simulink model "rf"  (R2016a)
settings: Solver=VariableStepAuto  StartTime=0.0  StopTime=10  RelTol=1e-3
values from neighbouring files (symbols this model uses):
  b_low_pass = fir1(low_pass_order, freq2rad(max_stop_freq_fir, fs), 'low', kaiser(low_pass_order+1, 0.5))    [graphs.m]    (also in rf_controller.m)
  band_pass_grpdelay = 10    [rf_controller.m]
  bandpass_a_H = bandpass_a_vec{i+M}    [rf_controller.m]
  bandpass_a_L = bandpass_a_vec{i}    [rf_controller.m]
  bandpass_b_H = bandpass_b_vec{i+M}    [rf_controller.m]
  bandpass_b_L = bandpass_b_vec{i}    [rf_controller.m]
  fs = 4224000    [bandpass_test.m]    (also in graphs.m = 50688000; main.m = 2*max_stop_freq_fir; rf_controller.m = 1/(time(2)-time(1)))
  LO2_sig = cos(2*pi*LO2 * time)    [rf_controller.m]
  low_pass_grpdelay = low_pass_order/2    (= 10)    [graphs.m]    (also in rf_controller.m)
  sig_len_band_pass = length(signal)/64    [rf_controller.m]
  sig_len_low_pass = length(signal)    [rf_controller.m]
undefined symbols (not defined in the file or in its folder): signal
libraries: dspsigops x5, lib1 x2
settings Model: Creator=jbeau  LastModifiedBy=jbeau
settings GRTTargetCC: GeneratePreprocessorConditionals=Use local settings

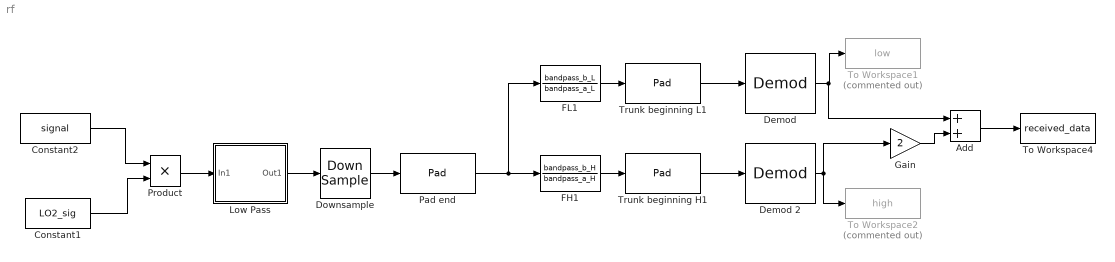
== system rf ==
  Add : Sum  OutDataTypeStr=double
  Constant1 : Constant  Value=LO2_sig  SampleTime=fs
  Constant2 : Constant  Value=signal  SampleTime=fs
  "Demod " : lib1/Demod 
  Demod 2 : lib1/Demod 
  Downsample : DownSample  N=64
  FH1 : DiscreteFilter  Numerator=bandpass_b_H  Denominator=bandpass_a_H  InputProcessing=Columns as channels (frame based)
  FL1 : DiscreteFilter  Numerator=bandpass_b_L  Denominator=bandpass_a_L  InputProcessing=Columns as channels (frame based)
  Gain : Gain  Gain=2
  Low Pass : Subsystem
  Pad end : dspsigops/Pad  padAlong=Columns  dimsToPad=1  valSrc=Specify via dialog  padVal=0  spec=Output size  padNumOutRowsSpecMethod=User-specified  numOutRows=sig_len_band_pass + band_pass_grpdelay  padNumOutColsSpecMethod=User-specified  numOutCols=1  isVarDimsMode=off  padBeginning=0  padEnd=0  outSizeMode=User-specified  outSize=1  padSigAt=End  trunc_flag=None  roundingMode=Floor  overflowMode=off  truncOrWrapMode=Truncate  wrap_flag=None
  Product : Product
  To Workspace1 : ToWorkspace  Commented=on  VariableName=low  SaveFormat=Timeseries  SampleTime=-1
  To Workspace2 : ToWorkspace  Commented=on  VariableName=high  SaveFormat=Timeseries  SampleTime=-1
  To Workspace4 : ToWorkspace  VariableName=received_data  SampleTime=-1
  Trunk beginning H1 : dspsigops/Pad  padAlong=Columns  dimsToPad=1  valSrc=Specify via dialog  padVal=0  spec=Output size  padNumOutRowsSpecMethod=User-specified  numOutRows=sig_len_band_pass  padNumOutColsSpecMethod=User-specified  numOutCols=1  isVarDimsMode=off  padBeginning=0  padEnd=0  outSizeMode=User-specified  outSize=1  padSigAt=Beginning  trunc_flag=None  roundingMode=Floor  overflowMode=off  truncOrWrapMode=Truncate  wrap_flag=None
  Trunk beginning L1 : dspsigops/Pad  padAlong=Columns  dimsToPad=1  valSrc=Specify via dialog  padVal=0  spec=Output size  padNumOutRowsSpecMethod=User-specified  numOutRows=sig_len_band_pass  padNumOutColsSpecMethod=User-specified  numOutCols=1  isVarDimsMode=off  padBeginning=0  padEnd=0  outSizeMode=User-specified  outSize=1  padSigAt=Beginning  trunc_flag=None  roundingMode=Floor  overflowMode=off  truncOrWrapMode=Truncate  wrap_flag=None
  wires:
  Constant1/1 -> Product/2
  Constant2/1 -> Product/1
  FL1/1 -> Trunk beginning L1/1
  FH1/1 -> Trunk beginning H1/1
  "Demod "/1 -> Add/1, To Workspace1/1
  Trunk beginning H1/1 -> Demod 2/1
  Trunk beginning L1/1 -> "Demod "/1
  Product/1 -> Low Pass/1(In1)
  Low Pass/1(Out1) -> Downsample/1
  Downsample/1 -> Pad end/1
  Pad end/1 -> FH1/1, FL1/1
  Demod 2/1 -> Gain/1, To Workspace2/1
  Gain/1 -> Add/2
  Add/1 -> To Workspace4/1

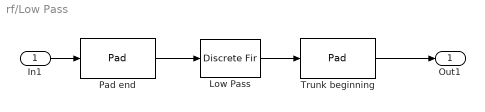
== system rf/Low Pass ==
  In1 : Inport
  "Low Pass " : DiscreteFir  Coefficients=b_low_pass  InputProcessing=Columns as channels (frame based)
  Pad end : dspsigops/Pad  padAlong=Columns  dimsToPad=1  valSrc=Specify via dialog  padVal=0  spec=Output size  padNumOutRowsSpecMethod=User-specified  numOutRows=sig_len_low_pass + low_pass_grpdelay  padNumOutColsSpecMethod=User-specified  numOutCols=1  isVarDimsMode=off  padBeginning=0  padEnd=0  outSizeMode=User-specified  outSize=1  padSigAt=End  trunc_flag=None  roundingMode=Floor  overflowMode=off  truncOrWrapMode=Truncate  wrap_flag=None
  Trunk beginning : dspsigops/Pad  padAlong=Columns  dimsToPad=1  valSrc=Specify via dialog  padVal=0  spec=Output size  padNumOutRowsSpecMethod=User-specified  numOutRows=sig_len_low_pass  padNumOutColsSpecMethod=User-specified  numOutCols=1  isVarDimsMode=off  padBeginning=0  padEnd=0  outSizeMode=User-specified  outSize=1  padSigAt=Beginning  trunc_flag=None  roundingMode=Floor  overflowMode=off  truncOrWrapMode=Truncate  wrap_flag=None
  Out1 : Outport
  wires:
  In1/1 -> Pad end/1
  Pad end/1 -> "Low Pass "/1
  "Low Pass "/1 -> Trunk beginning/1
  Trunk beginning/1 -> Out1/1
